simulink model "MinSegMega_Demo_V3"  (R2015a)
settings: Solver=FixedStepDiscrete  SolverMode=SingleTasking  StartTime=0.0  StopTime=inf  FixedStep=.05  RelTol=1e-3
libraries: arduinolib x9, MinSegLibrary_MinSegMega x4, RASPlib x2
settings Model: SimulationMode=external  ExtModeTrigDuration=2  Creator=Alec  LastModifiedBy=hurstj
settings OptimizationCC: ExpressionDepthLimit=2147483647  OptimizeModelRefInitCode=on  LifeSpan=1
settings DebuggingCC: UnderspecifiedInitializationDetection=Classic  MergeDetectMultiDrivingBlocksExec=none  StateNameClashWarn=warning
settings HardwareCC: ProdBitPerInt=16  ProdBitPerPointer=8  ProdIntDivRoundTo=Zero  ProdEndianess=LittleEndian  ProdWordSize=8  ProdHWDeviceType=Atmel->AVR
settings RTWCC: SystemTargetFile=realtime.tlc  GenerateMakefile=off  TemplateMakefile=realtime.tmf  Description=Real-Time Toolbox  RTWVerbose=off
settings CodeAppCC: CustomSymbolStrType=$N$R$M  InternalIdentifier=Classic
settings ERTTargetCC: CombineOutputUpdateFcns=off  ExtMode=on  ExtModeTransport=3  ExtModeMexArgs=0 45 115200 30  ERTSrcFileBannerTemplate=realtime_code_template.cgt  ERTHdrFileBannerTemplate=realtime_code_template.cgt  ERTDataSrcFileTemplate=realtime_code_template.cgt  ERTDataHdrFileTemplate=realtime_code_template.cgt  ERTCustomFileTemplate=realtime_file_process.tlc

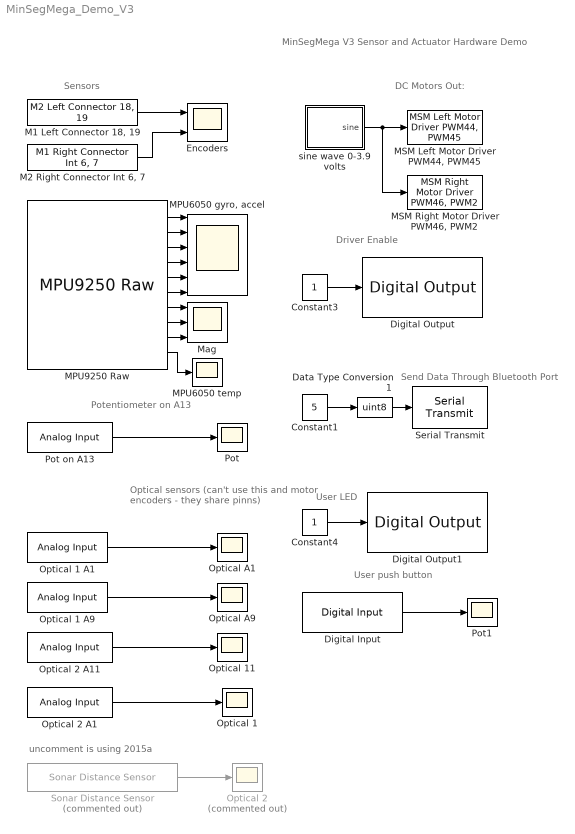
== system MinSegMega_Demo_V3 ==
  note: uncomment is using 2015a
  note: MinSegMega V3 Sensor and Actuator
      | Hardware Demo
  note: DC Motors Out:
  note: Sensors
  note: Send Data Through Bluetooth Port
  note: User push button
  note: Driver Enable
  note: Optical sensors (can't use this and
      | motor encoders - they share pinns)
  note: User LED
  note: Potentiometer on A13
  Constant1 : Constant  Value=5  SampleTime=-1
  Constant3 : Constant  SampleTime=-1
  Constant4 : Constant  SampleTime=-1
  Data Type Conversion1 : DataTypeConversion  OutDataTypeStr=uint8
  Digital Input : arduinolib/Digital Input  pinNumber=53  sampleTime=-1  blockPlatform=arduino
  Digital Output : arduinolib/Digital Output  pinNumber=42  blockPlatform=arduino
  Digital Output1 : arduinolib/Digital Output  pinNumber=49  blockPlatform=arduino
  Encoders : Scope  NumInputPorts=2
      settings: TimeRange=30  YMin=-6800~-191  YMax=-5750~-190
  "M1 Left Connector 18, 19" : MinSegLibrary_MinSegMega/M2 Left Connector 18, 19  Encoder=1  PinA=18  PinB=18
  "M2 Right Connector Int 6, 7" : MinSegLibrary_MinSegMega/M1 Right Connector Int 6, 7  Encoder=2  PinA=6  PinB=7
  "MPU6050 gyro, accel" : Scope  NumInputPorts=6
      settings: TimeRange=30  YMin=-10000~-5000~5000~-30000~-30000~-10000  YMax=12500~15000~27500~30000~30000~7500
  MPU6050 temp : Scope
      settings: TimeRange=30  YMin=1950  YMax=2350  SaveName=ScopeData2
  MPU9250 Raw : RASPlib/MPU9250 Raw  SimulateUsing=Code generation
  "MSM Left Motor Driver PWM44, PWM45" : MinSegLibrary_MinSegMega/MSM Left Motor Driver PWM44, PWM45  Vsupply=3.9  PWMoffset=0
  "MSM Right Motor Driver PWM46, PWM2 " : MinSegLibrary_MinSegMega/MSM Right Motor Driver PWM46, PWM2   Vsupply=3.9  PWMoffset=0
  Mag : Scope  NumInputPorts=3
      settings: TimeRange=30  YMin=-200~-200~-25  YMax=125~125~200  SaveName=ScopeData7
  Optical 1 : Scope
      settings: TimeRange=30  YMin=300  YMax=1100  SaveName=ScopeData8
  Optical 1 A1 : arduinolib/Analog Input  pinNumber=8  sampleTime=-1  blockPlatform=arduino
  Optical 1 A9 : arduinolib/Analog Input  pinNumber=9  sampleTime=-1  blockPlatform=arduino
  Optical 11 : Scope
      settings: TimeRange=30  YMin=300  YMax=1100  SaveName=ScopeData4
  Optical 2 : Scope  Commented=on
      settings: TimeRange=30  YMin=0  YMax=100  SaveName=ScopeData10
  Optical 2 A1 : arduinolib/Analog Input  pinNumber=12  sampleTime=-1  blockPlatform=arduino
  Optical 2 A11 : arduinolib/Analog Input  pinNumber=11  sampleTime=-1  blockPlatform=arduino
  Optical A1 : Scope
      settings: TimeRange=30  YMin=0  YMax=1000  SaveName=ScopeData9
  Optical A9 : Scope
      settings: TimeRange=30  YMin=0  YMax=1000  SaveName=ScopeData3
  Pot : Scope
      settings: TimeRange=30  YMin=0  YMax=1250  SaveName=ScopeData6
  Pot on A13 : arduinolib/Analog Input  pinNumber=13  sampleTime=-1  blockPlatform=arduino
  Pot1 : Scope
      settings: TimeRange=30  YMin=275  YMax=600  SaveName=ScopeData5
  Serial Transmit : arduinolib/Serial Transmit  portNumber=3  blockPlatform=arduino
  Sonar Distance Sensor : RASPlib/Sonar Distance Sensor  Commented=on  Sonar=1  TrigPin=16  EchoPin=17
  sine wave 0-3.9 volts : Subsystem
  wires:
  sine wave 0-3.9 volts/1(sine) -> "MSM Right Motor Driver PWM46, PWM2 "/1, "MSM Left Motor Driver PWM44, PWM45"/1
  Optical 1 A9/1 -> Optical A9/1
  Pot on A13/1 -> Pot/1
  Optical 2 A11/1 -> Optical 11/1
  Constant1/1 -> Data Type Conversion1/1
  Data Type Conversion1/1 -> Serial Transmit/1
  "M1 Left Connector 18, 19"/1 -> Encoders/1
  "M2 Right Connector Int 6, 7"/1 -> Encoders/2
  MPU9250 Raw/10 -> MPU6050 temp/1
  MPU9250 Raw/1 -> "MPU6050 gyro, accel"/1
  MPU9250 Raw/2 -> "MPU6050 gyro, accel"/2
  MPU9250 Raw/3 -> "MPU6050 gyro, accel"/3
  MPU9250 Raw/4 -> "MPU6050 gyro, accel"/4
  MPU9250 Raw/5 -> "MPU6050 gyro, accel"/5
  MPU9250 Raw/6 -> "MPU6050 gyro, accel"/6
  MPU9250 Raw/7 -> Mag/1
  MPU9250 Raw/8 -> Mag/2
  MPU9250 Raw/9 -> Mag/3
  Constant3/1 -> Digital Output/1
  Digital Input/1 -> Pot1/1
  Constant4/1 -> Digital Output1/1
  Optical 1 A1/1 -> Optical A1/1
  Optical 2 A1/1 -> Optical 1/1
  Sonar Distance Sensor/1 -> Optical 2/1

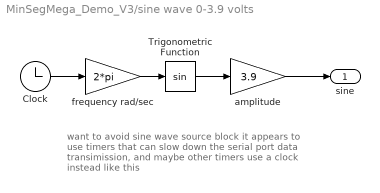
== system MinSegMega_Demo_V3/sine wave 0-3.9 volts ==
  note: want to avoid sine wave source block
      | it appears to use timers that can slow down the
      | serial port data transimission, and maybe
      | other timers
      |
      | use a clock instead like this
  Clock : Clock
  Trigonometric Function : Trigonometry
  amplitude : Gain  Gain=3.9
  frequency rad/sec : Gain  Gain=2*pi
  sine : Outport
  wires:
  amplitude/1 -> sine/1
  frequency rad/sec/1 -> Trigonometric Function/1
  Trigonometric Function/1 -> amplitude/1
  Clock/1 -> frequency rad/sec/1
